simulink model "AGC"  (R2024b)
settings: Solver=VariableStepAuto  StartTime=0.0  StopTime=10000  RelTol=1e-3
InitFcn:
  | Kl2=0.7;
  | Kl1=Kl2;
  | KPR=7;
  | B2=0.23;
  | B1=B2;
  | TG2=0.08;
  | TG1=TG2;
  | TT2=0.3;
  | TT1=TT2;
  | R2=2.4;
  | R1=R2;
  | Kp2=120;
  | Kp1=Kp2;
  | Tp2=20;
  | Tp1=Tp2;
  | T12=0.1*sqrt(3)/2;
  | PD2=1000;
  | PD1=5;
  | a12=0.9;
settings Model: Creator=86182  LastModifiedBy=86182

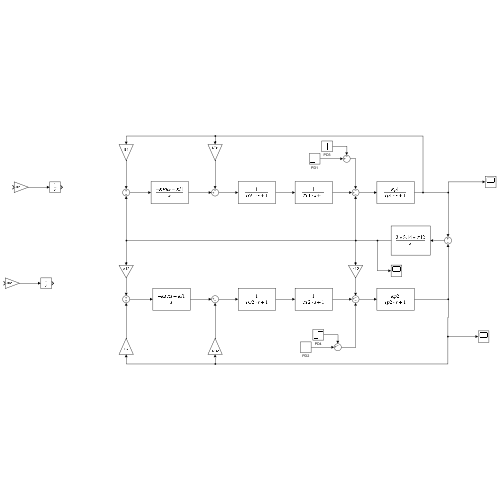
[thumbnail: Simulink's stored preview of the top-level diagram]
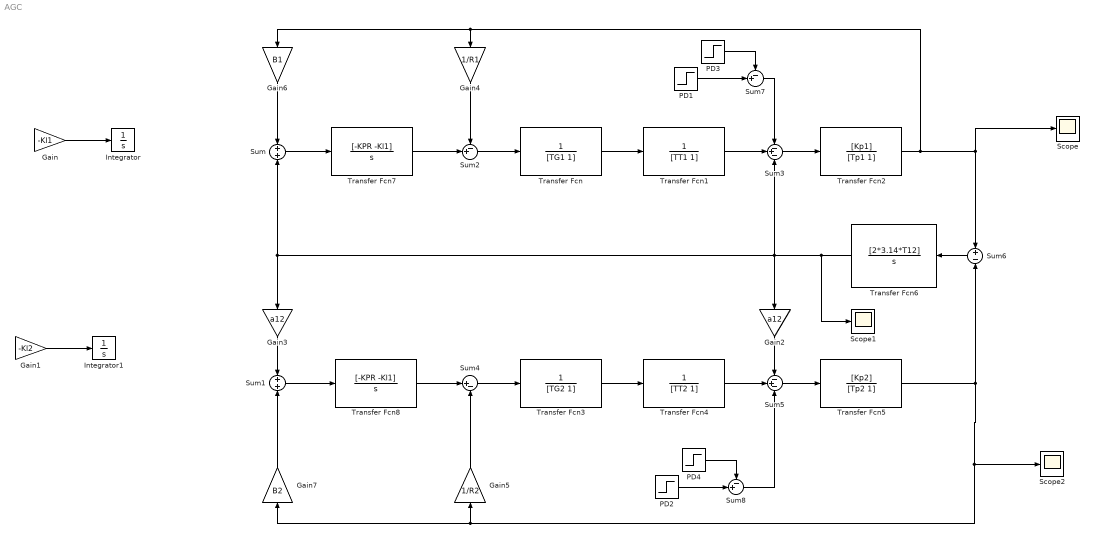
== system AGC ==
  Gain : Gain  Gain=-Kl1
  Gain1 : Gain  Gain=-Kl2
  Gain2 : Gain  Gain=a12
  Gain3 : Gain  Gain=a12
  Gain4 : Gain  Gain=1/R1
  Gain5 : Gain  Gain=1/R2
  Gain6 : Gain  Gain=B1
  Gain7 : Gain  Gain=B2
  Integrator : Integrator
  Integrator1 : Integrator
  PD1 : Step  Time=7  After=PD1  SampleTime=0
  PD2 : Step  Time=12  After=0  SampleTime=0
  PD3 : Step  Time=8  After=0  SampleTime=0
  PD4 : Step  Time=10  After=0  SampleTime=0
  Scope : Scope
  Scope1 : Scope
  Scope2 : Scope
  Sum : Sum  Inputs=+|+
  Sum1 : Sum  Inputs=+|+
  Sum2 : Sum  Inputs=-+|
  Sum3 : Sum  Inputs=-+-
  Sum4 : Sum  Inputs=|+-
  Sum5 : Sum  Inputs=-+-
  Sum6 : Sum  Inputs=+|-
  Sum7 : Sum  Inputs=-+|
  Sum8 : Sum  Inputs=-+|
  Transfer Fcn : TransferFcn  Denominator=[TG1 1]
  Transfer Fcn1 : TransferFcn  Denominator=[TT1 1]
  Transfer Fcn2 : TransferFcn  Numerator=[Kp1]  Denominator=[Tp1 1]
  Transfer Fcn3 : TransferFcn  Denominator=[TG2 1]
  Transfer Fcn4 : TransferFcn  Denominator=[TT2 1]
  Transfer Fcn5 : TransferFcn  Numerator=[Kp2]  Denominator=[Tp2 1]
  Transfer Fcn6 : TransferFcn  Numerator=[2*3.14*T12]  Denominator=[1 0]
  Transfer Fcn7 : TransferFcn  Numerator=[-KPR -Kl1]  Denominator=[1 0]
  Transfer Fcn8 : TransferFcn  Numerator=[-KPR -Kl1]  Denominator=[1 0]
  wires:
  Gain/1 -> Integrator/1
  Sum2/1 -> Transfer Fcn/1
  Transfer Fcn/1 -> Transfer Fcn1/1
  Transfer Fcn1/1 -> Sum3/2
  Sum3/1 -> Transfer Fcn2/1
  Transfer Fcn4/1 -> Sum5/2
  Gain1/1 -> Integrator1/1
  Sum5/1 -> Transfer Fcn5/1
  Sum4/1 -> Transfer Fcn3/1
  Transfer Fcn3/1 -> Transfer Fcn4/1
  Transfer Fcn2/1 -> Sum6/1, Scope/1, Gain6/1, Gain4/1
  Transfer Fcn5/1 -> Sum6/2, Gain7/1, Gain5/1, Scope2/1
  Gain3/1 -> Sum1/1
  Gain2/1 -> Sum5/1
  Gain4/1 -> Sum2/1
  Gain5/1 -> Sum4/2
  Gain6/1 -> Sum/1
  Gain7/1 -> Sum1/2
  Sum6/1 -> Transfer Fcn6/1
  Transfer Fcn6/1 -> Scope1/1, Sum/2, Gain3/1, Gain2/1, Sum3/3
  PD1/1 -> Sum7/2
  PD3/1 -> Sum7/1
  Sum7/1 -> Sum3/1
  PD4/1 -> Sum8/1
  PD2/1 -> Sum8/2
  Sum8/1 -> Sum5/3
  Sum/1 -> Transfer Fcn7/1
  Transfer Fcn7/1 -> Sum2/2
  Transfer Fcn8/1 -> Sum4/1
  Sum1/1 -> Transfer Fcn8/1
